simulink model "Full_Model_5"  (R2018b)
settings: Solver=VariableStepAuto  StartTime=0.0  StopTime=.5  RelTol=1e-3
InitFcn:
  | Robot_Body_Constants
values from neighbouring files (symbols this model uses):
  robot_radius = 0.0789    [Robot_Body_Constants.m]
  wheel_angles = [pi * 0.25 pi * 0.75 pi * 1.25 pi * 1.75]    [Robot_Body_Constants.m]
libraries: powerlib x56, peBldcCurrentController x4, simulink x1, dspinverses x1
(part 1 of 2)
settings Model: Creator=Zach  LastModifiedBy=Zach

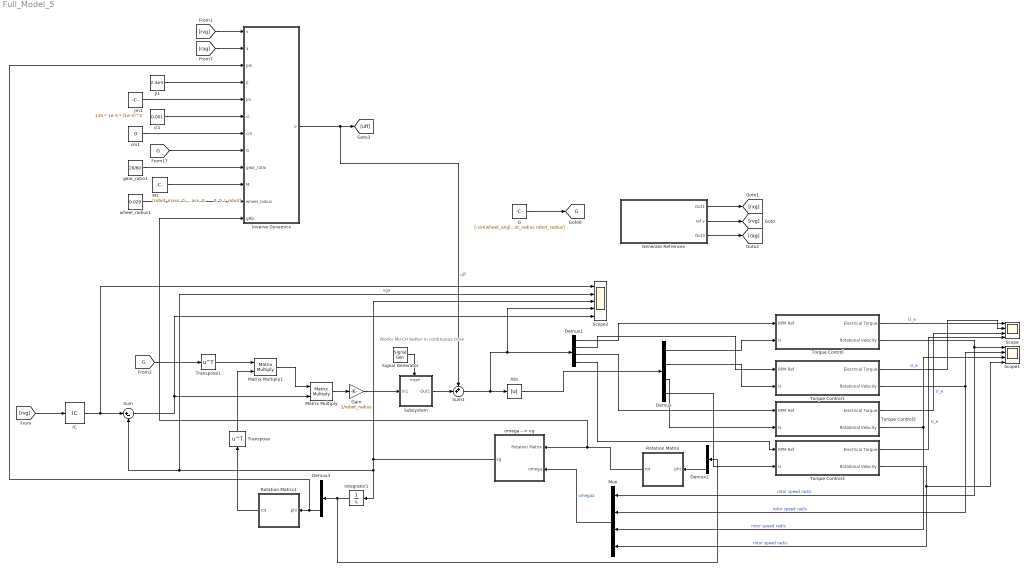
== system Full_Model_5 ==
  note: Works MUCH better in continuous time
  Abs : Abs
  Demux : Demux
  Demux1 : Demux
  Demux2 : Demux  Outputs=3
  Demux3 : Demux  Outputs=3
  G : Constant  Value=[-sin(wheel_angles(1)) -sin(wheel_angles(2)) -sin(wheel_angles(3)) -sin(wheel_angles(4)); cos(wheel_angles(1)) cos(wheel_angles(2)) cos(wheel_angles(3)) cos(wheel_angles(4)); robot_radius robot_radius robot_radius robot_radius]
  Gain : Gain  Gain=1/robot_radius
  Generate Refrences : Subsystem
  IC : InitialCondition  Value=[0;0;0]
  Integrator1 : Integrator
  Inverse Dynamics : MATLAB Function  TreatAsAtomicUnit=on
  Jl1 : Constant  Value=2.4e-5
  Jm1 : Constant  Value=135 * 1e-3 * (1e-2)^2
  M1 : Constant  Value=|
      | [robot_mass, 0, 0;
      |      0, robot_mass, 0;
      |      0, 0, I_robot]
  Matrix Multiply : Product  Multiplication=Matrix(*)
  Matrix Multiply1 : Product  Multiplication=Matrix(*)
  Mux : Mux
  Rotation Matrix : MATLAB Function  TreatAsAtomicUnit=on
  Rotation Matrix1 : MATLAB Function  TreatAsAtomicUnit=on
  Scope : Scope  NumInputPorts=4
  Scope1 : Scope  NumInputPorts=4
  Scope2 : Scope  NumInputPorts=5
  Signal Generator : SignalGenerator  Frequency=100000
  Subsystem : Subsystem
  Sum : Sum  Inputs=|+-
  Sum1 : Sum  Inputs=++|
  Torque Control : Subsystem
  Torque Control1 : Subsystem
  Torque Control2 : Subsystem
  Torque Control3 : Subsystem
  Transpose : Math  Operator=transpose  SaturateOnIntegerOverflow=on
  Transpose1 : Math  Operator=transpose  SaturateOnIntegerOverflow=on
  cl1 : Constant  Value=0.001
  cm1 : Constant  Value=0
  gear_ratio1 : Constant  Value=20/60
  omega --> vg : Subsystem
  wheel_radius1 : Constant  Value=0.029
  tag scope: G=global
  wires:
  Mux/1 -> omega --> vg/2(omega)  "omegaa"
  omega --> vg/1(vg) -> Scope2/3, Scope2/2, Sum/2, Integrator1/1  "vga"
  Generate Refrences/1(Out1) -> [rxg]
  Generate Refrences/2(ref v) -> [rvg]
  Generate Refrences/3(Out3) -> [rag]
  [rvg] -> IC/1
  Torque Control/2(Rotational Velocity) -> Mux/1, Scope1/1  "rotor speed rad/s"
  Torque Control/1(Electrical Torque) -> Scope/1  "U_e"
  Integrator1/1 -> Demux2/1, Demux3/1
  Demux2/3 -> Rotation Matrix/1(phi)
  G/1 -> [G]
  Rotation Matrix1/1(rot) -> Transpose/1
  [G] -> Transpose1/1
  Transpose/1 -> Matrix Multiply1/2
  IC/1 -> Scope2/1, Sum/1
  Sum/1 -> Scope2/5, Matrix Multiply/2
  Matrix Multiply1/1 -> Matrix Multiply/1
  Torque Control1/1(Electrical Torque) -> Scope/2  "U_e"
  Torque Control1/2(Rotational Velocity) -> Mux/2, Scope1/2  "rotor speed rad/s"
  Torque Control3/2(Rotational Velocity) -> Scope1/4, Mux/4  "rotor speed rad/s"
  Torque Control2/2(Rotational Velocity) -> Mux/3, Scope1/3  "rotor speed rad/s"
  Torque Control2/1(Electrical Torque) -> Scope/3  "U_e"
  Torque Control3/1(Electrical Torque) -> Scope/4  "U_e"
  Matrix Multiply/1 -> Gain/1
  Transpose1/1 -> Matrix Multiply1/1
  Abs/1 -> Demux/1
  Demux/4 -> Torque Control3/2(Is)
  Demux/1 -> Torque Control/2(Is)
  Demux/2 -> Torque Control1/2(Is)
  Demux/3 -> Torque Control2/2(Is)
  Demux1/1 -> Torque Control/1(RPM Ref)
  Demux1/2 -> Torque Control1/1(RPM Ref)
  Demux1/3 -> Torque Control2/1(RPM Ref)
  Demux1/4 -> Torque Control3/1(RPM Ref)
  gear_ratio1/1 -> Inverse Dynamics/9(gear_ratio)
  [G] -> Inverse Dynamics/8(G)
  Demux3/3 -> Inverse Dynamics/3(phi), Rotation Matrix1/1(phi)
  [rvg] -> Inverse Dynamics/1(v)
  cl1/1 -> Inverse Dynamics/6(cl)
  wheel_radius1/1 -> Inverse Dynamics/11(wheel_radius)
  cm1/1 -> Inverse Dynamics/7(cm)
  Inverse Dynamics/1(u) -> Sum1/1, [uff]  "uff"
  Jm1/1 -> Inverse Dynamics/5(Jm)
  [rag] -> Inverse Dynamics/2(a)
  Rotation Matrix/1(rot) -> Inverse Dynamics/12(gRb), omega --> vg/1(Rotation Matrix)
  Jl1/1 -> Inverse Dynamics/4(Jl)
  M1/1 -> Inverse Dynamics/10(M)
  Sum1/1 -> Scope2/4, Demux1/1, Abs/1
  Gain/1 -> Subsystem/1(In1)
  Subsystem/1(Out1) -> Sum1/2
  Signal Generator/1 -> Subsystem/Trigger

== system Full_Model_5/Generate Refrences ==
  Clock : Clock
  Constant : Constant  Value=3
  Gen Ref Values : MATLAB Function  TreatAsAtomicUnit=on
  Scope : Scope
  Out1 : Outport
  ref v : Outport  Port=2
  Out3 : Outport  Port=3
  wires:
  Clock/1 -> Scope/1, Gen Ref Values/2(t)
  Constant/1 -> Gen Ref Values/1(v)
  Gen Ref Values/1(rx) -> Out1/1
  Gen Ref Values/2(rv) -> ref v/1  "ref v"
  Gen Ref Values/3(ra) -> Out3/1

== system Full_Model_5/Subsystem ==
  In1 : Inport
  Trigger : TriggerPort  VariantControl=Variant  PortDimensions=1
  PID Controller : simulink/Continuous/PID Controller  Controller=PID  Form=Parallel  TimeDomain=Discrete-time  SampleTime=-1  IntegratorMethod=Forward Euler  FilterMethod=Forward Euler  ControllerParametersSource=internal  P=8  I=2  D=0  UseFilter=on  N=100  TunerSelectOption=Transfer Function Based (PID Tuner App)  InitialConditionSource=internal  InitialConditionForIntegrator=0  InitialConditionForFilter=0  DifferentiatorICPrevScaledInput=0  ExternalReset=none  TrackingMode=off  Kt=1  LimitOutput=on  UpperSaturationLimit=40  LowerSaturationLimit=-40  LinearizeAsGain=on  AntiWindupMode=none  Kb=1  POutMin=[]  POutMax=[]  IOutMin=[]  IOutMax=[]  DOutMin=[]  DOutMax=[]  NOutMin=[]  NOutMax=[]  SumOutMin=[]  SumOutMax=[]  SaturationOutMin=[]  SaturationOutMax=[]  PParamMin=[]  PParamMax=[]  IParamMin=[]  IParamMax=[]  DParamMin=[]  DParamMax=[]  NParamMin=[]  NParamMax=[]  KbParamMin=[]  KbParamMax=[]  KtParamMin=[]  KtParamMax=[]  KbOutMin=[]  KbOutMax=[]  KtOutMin=[]  KtOutMax=[]  IntegratorOutMin=[]  IntegratorOutMax=[]  FilterOutMin=[]  FilterOutMax=[]  SumI1OutMin=[]  SumI1OutMax=[]  SumI2OutMin=[]  SumI2OutMax=[]  SumI3OutMin=[]  SumI3OutMax=[]  SumI4OutMin=[]  SumI4OutMax=[]  SumDOutMin=[]  SumDOutMax=[]  DifferentiatorOutMin=[]  DifferentiatorOutMax=[]  FilterDiffOutCoefMin=[]  FilterDiffOutCoefMax=[]  ReciprocalOutMin=[]  ReciprocalOutMax=[]  SumDenOutMin=[]  SumDenOutMax=[]  SumNumOutMin=[]  SumNumOutMax=[]  DivideOutMin=[]  DivideOutMax=[]  IntegratorContinuousStateAttributes=''  IntegratorStateMustResolveToSignalObject=off  IntegratorRTWStateStorageClass=Auto  FilterContinuousStateAttributes=''  FilterStateMustResolveToSignalObject=off  FilterRTWStateStorageClass=Auto  ParallelPVariant=InternalParameters  IdealPVariant=Disabled  IVariant=InternalParameters  DVariant=InternalParameters  IntegratorVariant=Discrete  SatVariant=Enabled  AWVariant=Passthrough  PCopyVariant=Disabled  TRVariant=Disabled  FdbkBlocksVariant=Forward  IdealPFdbkVariant=Disabled  SatFdbkVariant=Disabled  DerivativeFilterVariant=ForwardEulerFilter  NVariant=InternalParameters  NCopyVariant=Disabled  FilterICVariant=InternalICsFilter  IntegratorICVariant=InternalICs  ExternalResetVariant=Disabled  TRSumVariant=Passthrough  SumFdbkVariant=Disabled  SumVariant=Sum_PID
  Out1 : Outport
  wires:
  In1/1 -> PID Controller/1
  PID Controller/1 -> Out1/1

== system Full_Model_5/Torque Control ==
  note: Needed for direction
  RPM Ref : Inport
  Is : Inport  Port=2
  Subsystem : Subsystem
  Subsystem1 : Subsystem
  Electrical Torque : Outport
  Rotational Velocity : Outport  Port=2
  wires:
  Subsystem/1(Gating Signals (PWM)) -> Subsystem1/1(Gating Signals)
  RPM Ref/1 -> Subsystem/1(rpm ref)
  Is/1 -> Subsystem/2(Is*)
  Subsystem1/2(Omega) -> Rotational Velocity/1
  Subsystem1/1(Te) -> Electrical Torque/1
  Subsystem1/3(Iabc) -> Subsystem/3(Iabc)
  Subsystem1/4(Out1) -> Subsystem/4(H1)
  Subsystem1/5(Out2) -> Subsystem/5(H2)
  Subsystem1/6(Out3) -> Subsystem/6(H3)

== system Full_Model_5/Torque Control1 ==
  note: Needed for direction
  RPM Ref : Inport
  Is : Inport  Port=2
  Subsystem : Subsystem
  Subsystem1 : Subsystem
  Electrical Torque : Outport
  Rotational Velocity : Outport  Port=2
  wires:
  Subsystem1/6(Out3) -> Subsystem/6(H3)
  Subsystem1/5(Out2) -> Subsystem/5(H2)
  Subsystem1/4(Out1) -> Subsystem/4(H1)
  Subsystem1/3(Iabc) -> Subsystem/3(Iabc)
  Subsystem1/1(Te) -> Electrical Torque/1
  Subsystem1/2(Omega) -> Rotational Velocity/1
  Is/1 -> Subsystem/2(Is*)
  RPM Ref/1 -> Subsystem/1(rpm ref)
  Subsystem/1(Gating Signals (PWM)) -> Subsystem1/1(Gating Signals)

== system Full_Model_5/Torque Control2 ==
  note: Needed for direction
  RPM Ref : Inport
  Is : Inport  Port=2
  Subsystem : Subsystem
  Subsystem1 : Subsystem
  Electrical Torque : Outport
  Rotational Velocity : Outport  Port=2
  wires:
  Subsystem/1(Gating Signals (PWM)) -> Subsystem1/1(Gating Signals)
  RPM Ref/1 -> Subsystem/1(rpm ref)
  Is/1 -> Subsystem/2(Is*)
  Subsystem1/2(Omega) -> Rotational Velocity/1
  Subsystem1/1(Te) -> Electrical Torque/1
  Subsystem1/3(Iabc) -> Subsystem/3(Iabc)
  Subsystem1/4(Out1) -> Subsystem/4(H1)
  Subsystem1/5(Out2) -> Subsystem/5(H2)
  Subsystem1/6(Out3) -> Subsystem/6(H3)

== system Full_Model_5/Torque Control3 ==
  note: Needed for direction
  RPM Ref : Inport
  Is : Inport  Port=2
  Subsystem : Subsystem
  Subsystem1 : Subsystem
  Electrical Torque : Outport
  Rotational Velocity : Outport  Port=2
  wires:
  Subsystem1/6(Out3) -> Subsystem/6(H3)
  Subsystem1/5(Out2) -> Subsystem/5(H2)
  Subsystem1/4(Out1) -> Subsystem/4(H1)
  Subsystem1/3(Iabc) -> Subsystem/3(Iabc)
  Subsystem1/1(Te) -> Electrical Torque/1
  Subsystem1/2(Omega) -> Rotational Velocity/1
  Is/1 -> Subsystem/2(Is*)
  RPM Ref/1 -> Subsystem/1(rpm ref)
  Subsystem/1(Gating Signals (PWM)) -> Subsystem1/1(Gating Signals)

== system Full_Model_5/omega --> vg ==
  Rotation Matrix : Inport
  omega : Inport  Port=2
  Gain : Gain  Gain=robot_radius
  Matrix Multiply : Product  Inputs=3  Multiplication=Matrix(*)
  Pseudoinverse : dspinverses/Pseudoinverse  wanterr=off  SimulateUsing=Interpreted execution
      settings: SourceProductName=DSP System Toolbox  SourceProductBaseCode=DS
  Transpose : Math  Operator=transpose  SaturateOnIntegerOverflow=on
  vg : Outport
  wires:
  [G] -> Transpose/1
  Transpose/1 -> Pseudoinverse/1
  omega/1 -> Matrix Multiply/3
  Matrix Multiply/1 -> Gain/1
  Gain/1 -> vg/1
  Pseudoinverse/1 -> Matrix Multiply/2
  Rotation Matrix/1 -> Matrix Multiply/1

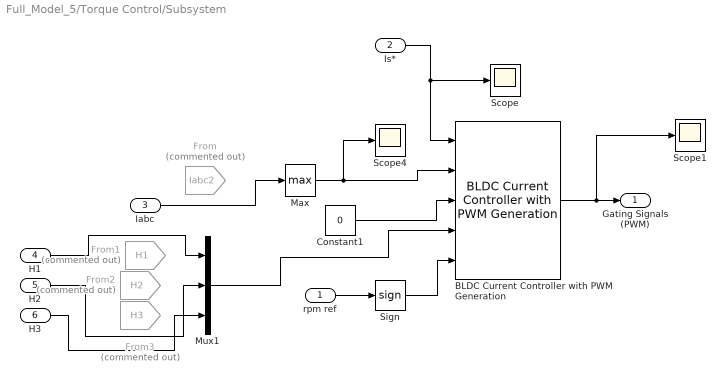
== system Full_Model_5/Torque Control/Subsystem ==
  rpm ref : Inport
  Is* : Inport  Port=2
  Iabc : Inport  Port=3
  H1 : Inport  Port=4
  H2 : Inport  Port=5
  H3 : Inport  Port=6
  BLDC Current Controller with PWM Generation : peBldcCurrentController/BLDC Current Controller with PWM Generation  Kp=40  Ki=10  Kaw=100  Ts=-1  Tsd=0.001  ActZC=off  CarrCount=Up  Tper=.0001  Tfundamental=.00001
  Constant1 : Constant  Value=0
  From : From  Commented=on  GotoTag=Iabc2  TagVisibility=global
  From1 : From  Commented=on  GotoTag=H1  TagVisibility=global
  From2 : From  Commented=on  GotoTag=H2  TagVisibility=global
  From3 : From  Commented=on  GotoTag=H3  TagVisibility=global
  Max : MinMax  Function=max
  Mux1 : Mux  Inputs=3
  Scope : Scope
  Scope1 : Scope
  Scope4 : Scope
  Sign : Signum
  Gating Signals (PWM) : Outport
  wires:
  rpm ref/1 -> Sign/1
  Mux1/1 -> BLDC Current Controller with PWM Generation/4
  Sign/1 -> BLDC Current Controller with PWM Generation/5
  Constant1/1 -> BLDC Current Controller with PWM Generation/3
  Max/1 -> BLDC Current Controller with PWM Generation/2, Scope4/1
  BLDC Current Controller with PWM Generation/1 -> Scope1/1, Gating Signals (PWM)/1
  Is*/1 -> Scope/1, BLDC Current Controller with PWM Generation/1
  Iabc/1 -> Max/1
  H1/1 -> Mux1/1
  H2/1 -> Mux1/2
  H3/1 -> Mux1/3

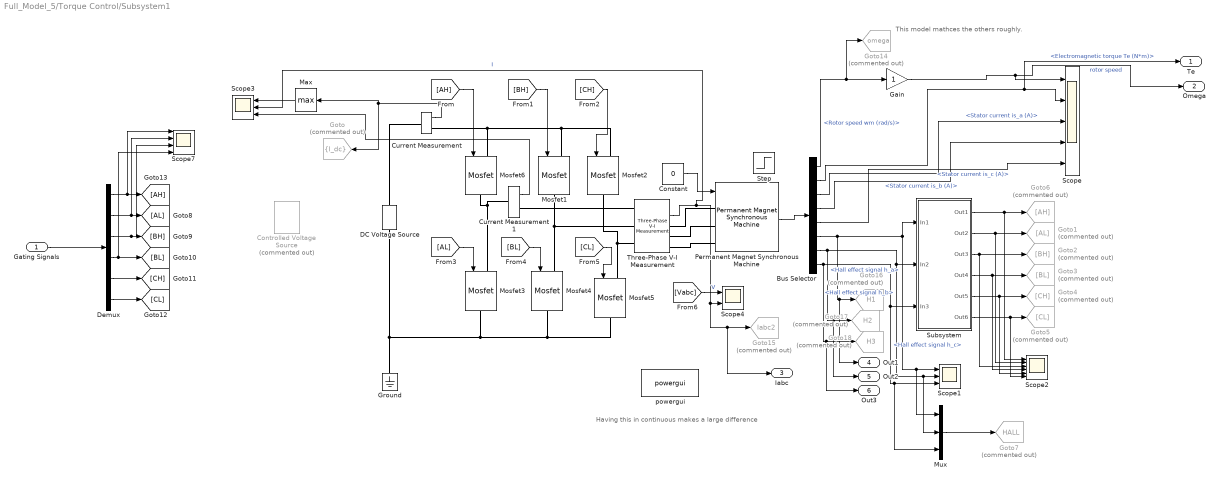
== system Full_Model_5/Torque Control/Subsystem1 ==
  note: This model mathces the others roughly.
  note: Having this in continuous makes a large difference
  Gating Signals : Inport
  Bus Selector : BusSelector  OutputSignals=Rotor speed wm (rad/s),Electromagnetic torque Te (N*m),Stator current is_a (A),Stator current is_b (A),Stator current is_c (A),Hall effect signal h_a,Hall effect signal h_b,Hall effect signal h_c
  Constant : Constant  Value=0
  Controlled Voltage Source : powerlib/Electrical Sources/Controlled Voltage Source  Commented=on  Initialize=off  Source_Type=DC  Amplitude=24  Phase=0  Frequency=0  Measurements=Voltage
  Current Measurement : powerlib/Measurements/Current Measurement  PhasorSimulation=off  OutputType=Magnitude  PSBequivalent=0
  Current Measurement1 : powerlib/Measurements/Current Measurement  PhasorSimulation=off  OutputType=Complex  PSBequivalent=0
  DC Voltage Source : powerlib/Electrical Sources/DC Voltage Source  Amplitude=24  Measurements=None
  Demux : Demux  Outputs=6
  Gain : Gain
  Goto : Goto  Commented=on  GotoTag=I_dc  TagVisibility=scoped
  Goto1 : Goto  Commented=on  GotoTag=AL
  Goto14 : Goto  Commented=on  GotoTag=omega  TagVisibility=global
  Goto15 : Goto  Commented=on  GotoTag=Iabc2  TagVisibility=global
  Goto16 : Goto  Commented=on  GotoTag=H1  TagVisibility=global
  Goto17 : Goto  Commented=on  GotoTag=H2  TagVisibility=global
  Goto18 : Goto  Commented=on  GotoTag=H3  TagVisibility=global
  Goto2 : Goto  Commented=on  GotoTag=BH
  Goto3 : Goto  Commented=on  GotoTag=BL
  Goto4 : Goto  Commented=on  GotoTag=CH
  Goto5 : Goto  Commented=on  GotoTag=CL
  Goto6 : Goto  Commented=on  GotoTag=AH
  Goto7 : Goto  Commented=on  GotoTag=HALL  TagVisibility=global
  Ground : powerlib/Elements/Ground  LConnTagsString=a
  Max : MinMax  Function=max
  Mosfet{1..6} (6 alike) : powerlib/Power Electronics/Mosfet  Ron=0.1  Lon=0  Rd=0.01  Vfd=0  IC=0  Rs=1e5  Cs=inf  Measurements=off
  Mux : Mux  Inputs=3
  Permanent Magnet Synchronous Machine : powerlib/Machines/Permanent Magnet Synchronous Machine  NbPhases=3  FluxDistribution=Trapezoidal  RotorType=Round  MechanicalLoad=Torque Tm  PresetModel=No  ShowDetailedParameters=on  MeasurementBus=off  Resistance=0.304  Inductance=0.0002315  dqInductances=[8.5e-3,8.5e-3]  La=0.0002315  MachineConstant=Torque Constant (N.m / A_peak)  Flux=0.003258  VoltageCst=5.4588  TorqueCst=0.052128  Flat=120  Mechanical=[1.81e-05 1e-07 8]  PolePairs=4  InitialConditions=[0,0, 0,0]  InitialConditions5ph=[0 0 0 0 0 0]  TsPowergui=0  TsBlock=-1  RefAngle=Aligned with phase A axis (original Park)
      settings: SourceProductName=Simscape Power Systems
  Scope : Scope  NumInputPorts=5
  Scope1 : Scope  NumInputPorts=3
  Scope2 : Scope  NumInputPorts=6
  Scope3 : Scope  NumInputPorts=3
  Scope4 : Scope  NumInputPorts=2
  Scope7 : Scope  NumInputPorts=4
  Step : Step  Time=.1  After=.125  SampleTime=0
  Subsystem : Subsystem
  Three-Phase V-I Measurement : powerlib/Measurements/Three-Phase V-I Measurement  VoltageMeasurement=phase-to-ground  SetLabelV=off  LabelV=Vabc  Vpu=off  VpuLL=off  CurrentMeasurement=yes  SetLabelI=off  LabelI=Iabc  Ipu=off  Pbase=100e6  Vbase=500e3  OutputType=Complex  PhasorSimulation=off  PSBequivalent=0
  powergui : powerlib/powergui  Priority=1  SimulationMode=Continuous  SampleTime=50e-6  frequency=60  Iterations=50  frequencyindice=0  Pbase=100e6  ErrMax=1e-4  UnitsV=kV  UnitsW=MW  buscounter=0  FunctionMessages=off  echomessages=off  EnableUseOfTLC=off  CurrentSourceSwitches=off  DisableSnubberDevices=off  DisableRonSwitches=off  DisableVfSwitches=off  DisplayEquations=off  SolverType=Tustin/Backward Euler (TBE)  Interpol=off  ExternalGateDelay=off  methode=off  Ts=100  x0status=blocks  SPID=on  SwTol=0  HookPort=off  RestoreLinks=warning  ResistiveCurrentMeasurement=off  Frange=[0:2:500]  Ylog=off  Xlog=on  ShowGrid=off  save=off  variable=ZData  structure=0  ZoomFFT=off  StartTime=0.0  cycles=1  DisplayStyle=1  fundamental=60  FreqAxis=off  MaxFrequency=1000  frequencyindicesteady=1  RmsSteady=1  display=off
  Te : Outport
  Omega : Outport  Port=2
  Iabc : Outport  Port=3
  Out1 : Outport  Port=4
  Out2 : Outport  Port=5
  Out3 : Outport  Port=6
  wires:
  [CH] -> Mosfet2/1
  Subsystem/6(Out6) -> Scope2/6, Goto5/1
  Subsystem/2(Out2) -> Scope2/2, Goto1/1
  Bus Selector/8 -> Out3/1, Goto18/1, Mux/3, Scope1/3, Subsystem/3(In3)  "<Hall effect signal h_c>"
  Subsystem/1(Out1) -> Scope2/1, Goto6/1
  Subsystem/3(Out3) -> Scope2/3, Goto2/1
  Bus Selector/2 -> Te/1, Scope/2  "<Electromagnetic torque Te (N*m)>"
  Subsystem/4(Out4) -> Scope2/4, Goto3/1
  Bus Selector/1 -> Goto14/1, Gain/1  "<Rotor speed wm (rad/s)>"
  Bus Selector/7 -> Out2/1, Goto17/1, Mux/2, Scope1/2, Subsystem/2(In2)  "<Hall effect signal h_b>"
  Mux/1 -> Goto7/1
  [AL] -> Mosfet3/1
  [BL] -> Mosfet4/1
  Bus Selector/6 -> Out1/1, Goto16/1, Subsystem/1(In1), Mux/1, Scope1/1  "<Hall effect signal h_a>"
  Subsystem/5(Out5) -> Scope2/5, Goto4/1
  [CL] -> Mosfet5/1
  Current Measurement/1 -> Max/1, Goto/1
  Bus Selector/3 -> Scope/3  "<Stator current is_a (A)>"
  Permanent Magnet Synchronous Machine/1 -> Bus Selector/1
  [BH] -> Mosfet1/1
  [AH] -> Mosfet6/1
  Bus Selector/4 -> Scope/4  "<Stator current is_b (A)>"
  Gain/1 -> Omega/1, Scope/1  "rotor speed"
  Bus Selector/5 -> Scope/5  "<Stator current is_c (A)>"
  Demux/6 -> [CL]
  Demux/5 -> [CH]
  Demux/4 -> [BL], Scope7/4
  Demux/3 -> Scope7/3, [BH]
  Demux/2 -> Scope7/2, [AL]
  Demux/1 -> Scope7/1, [AH]
  [Vabc] -> Scope4/1  "V"
  Three-Phase V-I Measurement/2 -> Iabc/1, Goto15/1, Scope4/2, Scope3/2  "I"
  Gating Signals/1 -> Demux/1
  Max/1 -> Scope3/1
  Current Measurement1/1 -> Scope3/3
  Constant/1 -> Permanent Magnet Synchronous Machine/1
  connections:
  Mosfet1/RConn1 -- Three-Phase V-I Measurement/LConn2 -- Mosfet4/LConn1
  Mosfet2/RConn1 -- Three-Phase V-I Measurement/LConn3 -- Mosfet5/LConn1
  Mosfet6/RConn1 -- Current Measurement1/LConn1 -- Mosfet3/LConn1
  Mosfet6/LConn1 -- Current Measurement/RConn1 -- Mosfet2/LConn1 -- Mosfet1/LConn1
  Ground/LConn1 -- DC Voltage Source/LConn1 -- Mosfet5/RConn1 -- Mosfet4/RConn1 -- Mosfet3/RConn1
  Three-Phase V-I Measurement/RConn1 -- Permanent Magnet Synchronous Machine/LConn1
  Three-Phase V-I Measurement/RConn2 -- Permanent Magnet Synchronous Machine/LConn2
  Permanent Magnet Synchronous Machine/LConn3 -- Three-Phase V-I Measurement/RConn3
  DC Voltage Source/RConn1 -- Current Measurement/LConn1
  Current Measurement1/RConn1 -- Three-Phase V-I Measurement/LConn1

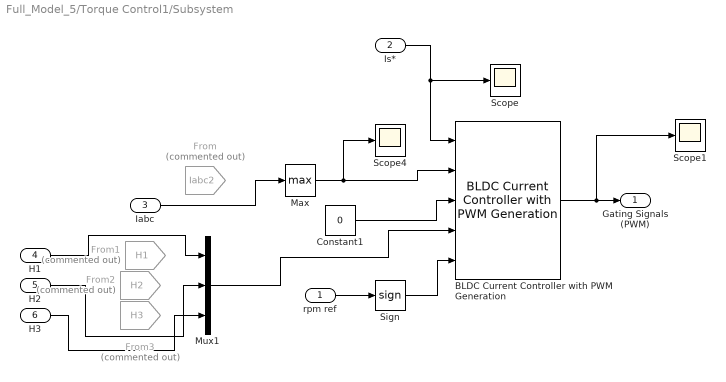
== system Full_Model_5/Torque Control1/Subsystem ==
  rpm ref : Inport
  Is* : Inport  Port=2
  Iabc : Inport  Port=3
  H1 : Inport  Port=4
  H2 : Inport  Port=5
  H3 : Inport  Port=6
  BLDC Current Controller with PWM Generation : peBldcCurrentController/BLDC Current Controller with PWM Generation  Kp=40  Ki=10  Kaw=100  Ts=-1  Tsd=0.001  ActZC=off  CarrCount=Up  Tper=.0001  Tfundamental=.00001
  Constant1 : Constant  Value=0
  From : From  Commented=on  GotoTag=Iabc2  TagVisibility=global
  From1 : From  Commented=on  GotoTag=H1  TagVisibility=global
  From2 : From  Commented=on  GotoTag=H2  TagVisibility=global
  From3 : From  Commented=on  GotoTag=H3  TagVisibility=global
  Max : MinMax  Function=max
  Mux1 : Mux  Inputs=3
  Scope : Scope
  Scope1 : Scope
  Scope4 : Scope
  Sign : Signum
  Gating Signals (PWM) : Outport
  wires:
  H3/1 -> Mux1/3
  H2/1 -> Mux1/2
  H1/1 -> Mux1/1
  Iabc/1 -> Max/1
  Is*/1 -> BLDC Current Controller with PWM Generation/1, Scope/1
  BLDC Current Controller with PWM Generation/1 -> Gating Signals (PWM)/1, Scope1/1
  Max/1 -> Scope4/1, BLDC Current Controller with PWM Generation/2
  Constant1/1 -> BLDC Current Controller with PWM Generation/3
  Sign/1 -> BLDC Current Controller with PWM Generation/5
  Mux1/1 -> BLDC Current Controller with PWM Generation/4
  rpm ref/1 -> Sign/1

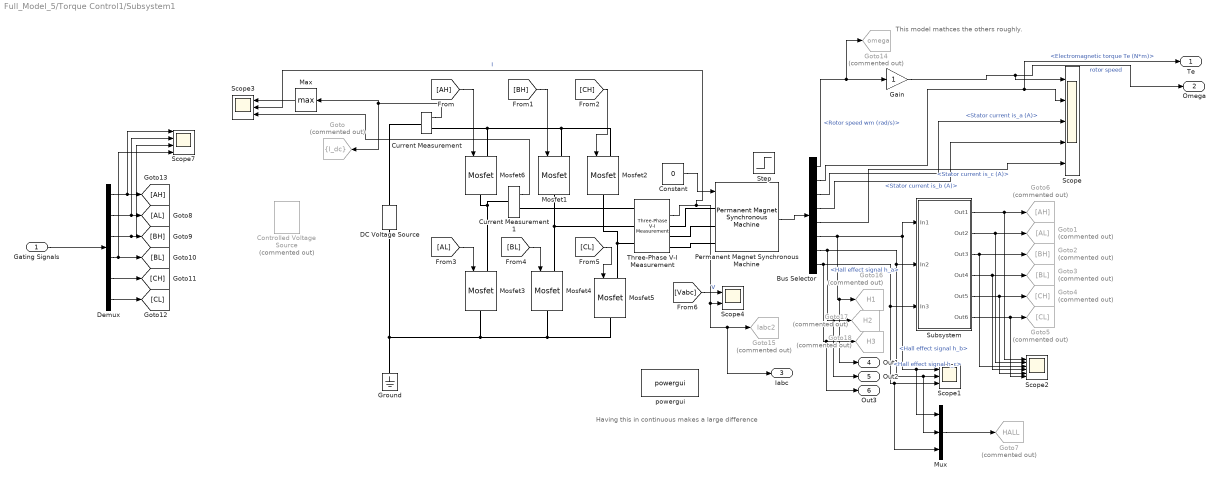
== system Full_Model_5/Torque Control1/Subsystem1 ==
  note: Having this in continuous makes a large difference
  note: This model mathces the others roughly.
  Gating Signals : Inport
  Bus Selector : BusSelector  OutputSignals=Rotor speed wm (rad/s),Electromagnetic torque Te (N*m),Stator current is_a (A),Stator current is_b (A),Stator current is_c (A),Hall effect signal h_a,Hall effect signal h_b,Hall effect signal h_c
  Constant : Constant  Value=0
  Controlled Voltage Source : powerlib/Electrical Sources/Controlled Voltage Source  Commented=on  Initialize=off  Source_Type=DC  Amplitude=24  Phase=0  Frequency=0  Measurements=Voltage
  Current Measurement : powerlib/Measurements/Current Measurement  PhasorSimulation=off  OutputType=Magnitude  PSBequivalent=0
  Current Measurement1 : powerlib/Measurements/Current Measurement  PhasorSimulation=off  OutputType=Complex  PSBequivalent=0
  DC Voltage Source : powerlib/Electrical Sources/DC Voltage Source  Amplitude=24  Measurements=None
  Demux : Demux  Outputs=6
  Gain : Gain
  Goto : Goto  Commented=on  GotoTag=I_dc  TagVisibility=scoped
  Goto1 : Goto  Commented=on  GotoTag=AL
  Goto14 : Goto  Commented=on  GotoTag=omega  TagVisibility=global
  Goto15 : Goto  Commented=on  GotoTag=Iabc2  TagVisibility=global
  Goto16 : Goto  Commented=on  GotoTag=H1  TagVisibility=global
  Goto17 : Goto  Commented=on  GotoTag=H2  TagVisibility=global
  Goto18 : Goto  Commented=on  GotoTag=H3  TagVisibility=global
  Goto2 : Goto  Commented=on  GotoTag=BH
  Goto3 : Goto  Commented=on  GotoTag=BL
  Goto4 : Goto  Commented=on  GotoTag=CH
  Goto5 : Goto  Commented=on  GotoTag=CL
  Goto6 : Goto  Commented=on  GotoTag=AH
  Goto7 : Goto  Commented=on  GotoTag=HALL  TagVisibility=global
  Ground : powerlib/Elements/Ground  LConnTagsString=a
  Max : MinMax  Function=max
  Mosfet{1..6} (6 alike) : powerlib/Power Electronics/Mosfet  Ron=0.1  Lon=0  Rd=0.01  Vfd=0  IC=0  Rs=1e5  Cs=inf  Measurements=off
  Mux : Mux  Inputs=3
  Permanent Magnet Synchronous Machine : powerlib/Machines/Permanent Magnet Synchronous Machine  NbPhases=3  FluxDistribution=Trapezoidal  RotorType=Round  MechanicalLoad=Torque Tm  PresetModel=No  ShowDetailedParameters=on  MeasurementBus=off  Resistance=0.304  Inductance=0.0002315  dqInductances=[8.5e-3,8.5e-3]  La=0.0002315  MachineConstant=Torque Constant (N.m / A_peak)  Flux=0.003258  VoltageCst=5.4588  TorqueCst=0.052128  Flat=120  Mechanical=[1.81e-05 1e-07 8]  PolePairs=4  InitialConditions=[0,0, 0,0]  InitialConditions5ph=[0 0 0 0 0 0]  TsPowergui=0  TsBlock=-1  RefAngle=Aligned with phase A axis (original Park)
      settings: SourceProductName=Simscape Power Systems
  Scope : Scope  NumInputPorts=5
  Scope1 : Scope  NumInputPorts=3
  Scope2 : Scope  NumInputPorts=6
  Scope3 : Scope  NumInputPorts=3
  Scope4 : Scope  NumInputPorts=2
  Scope7 : Scope  NumInputPorts=4
  Step : Step  Time=.1  After=.125  SampleTime=0
  Subsystem : Subsystem
  Three-Phase V-I Measurement : powerlib/Measurements/Three-Phase V-I Measurement  VoltageMeasurement=phase-to-ground  SetLabelV=off  LabelV=Vabc  Vpu=off  VpuLL=off  CurrentMeasurement=yes  SetLabelI=off  LabelI=Iabc  Ipu=off  Pbase=100e6  Vbase=500e3  OutputType=Complex  PhasorSimulation=off  PSBequivalent=0
  powergui : powerlib/powergui  Priority=1  SimulationMode=Continuous  SampleTime=50e-6  frequency=60  Iterations=50  frequencyindice=0  Pbase=100e6  ErrMax=1e-4  UnitsV=kV  UnitsW=MW  buscounter=0  FunctionMessages=off  echomessages=off  EnableUseOfTLC=off  CurrentSourceSwitches=off  DisableSnubberDevices=off  DisableRonSwitches=off  DisableVfSwitches=off  DisplayEquations=off  SolverType=Tustin/Backward Euler (TBE)  Interpol=off  ExternalGateDelay=off  methode=off  Ts=100  x0status=blocks  SPID=on  SwTol=0  HookPort=off  RestoreLinks=warning  ResistiveCurrentMeasurement=off  Frange=[0:2:500]  Ylog=off  Xlog=on  ShowGrid=off  save=off  variable=ZData  structure=0  ZoomFFT=off  StartTime=0.0  cycles=1  DisplayStyle=1  fundamental=60  FreqAxis=off  MaxFrequency=1000  frequencyindicesteady=1  RmsSteady=1  display=off
  Te : Outport
  Omega : Outport  Port=2
  Iabc : Outport  Port=3
  Out1 : Outport  Port=4
  Out2 : Outport  Port=5
  Out3 : Outport  Port=6
  wires:
  Constant/1 -> Permanent Magnet Synchronous Machine/1
  Current Measurement1/1 -> Scope3/3
  Max/1 -> Scope3/1
  Gating Signals/1 -> Demux/1
  Three-Phase V-I Measurement/2 -> Scope3/2, Scope4/2, Goto15/1, Iabc/1  "I"
  [Vabc] -> Scope4/1  "V"
  Demux/1 -> [AH], Scope7/1
  Demux/2 -> [AL], Scope7/2
  Demux/3 -> [BH], Scope7/3
  Demux/4 -> Scope7/4, [BL]
  Demux/5 -> [CH]
  Demux/6 -> [CL]
  Bus Selector/5 -> Scope/5  "<Stator current is_c (A)>"
  Gain/1 -> Scope/1, Omega/1  "rotor speed"
  Bus Selector/4 -> Scope/4  "<Stator current is_b (A)>"
  [AH] -> Mosfet6/1
  [BH] -> Mosfet1/1
  Permanent Magnet Synchronous Machine/1 -> Bus Selector/1
  Bus Selector/3 -> Scope/3  "<Stator current is_a (A)>"
  Current Measurement/1 -> Goto/1, Max/1
  [CL] -> Mosfet5/1
  Subsystem/5(Out5) -> Goto4/1, Scope2/5
  Bus Selector/6 -> Scope1/1, Mux/1, Subsystem/1(In1), Goto16/1, Out1/1  "<Hall effect signal h_a>"
  [BL] -> Mosfet4/1
  [AL] -> Mosfet3/1
  Mux/1 -> Goto7/1
  Bus Selector/7 -> Subsystem/2(In2), Scope1/2, Mux/2, Goto17/1, Out2/1  "<Hall effect signal h_b>"
  Bus Selector/1 -> Gain/1, Goto14/1  "<Rotor speed wm (rad/s)>"
  Subsystem/4(Out4) -> Goto3/1, Scope2/4
  Bus Selector/2 -> Scope/2, Te/1  "<Electromagnetic torque Te (N*m)>"
  Subsystem/3(Out3) -> Goto2/1, Scope2/3
  Subsystem/1(Out1) -> Goto6/1, Scope2/1
  Bus Selector/8 -> Subsystem/3(In3), Scope1/3, Mux/3, Goto18/1, Out3/1  "<Hall effect signal h_c>"
  Subsystem/2(Out2) -> Goto1/1, Scope2/2
  Subsystem/6(Out6) -> Goto5/1, Scope2/6
  [CH] -> Mosfet2/1
  connections:
  Current Measurement1/RConn1 -- Three-Phase V-I Measurement/LConn1
  DC Voltage Source/RConn1 -- Current Measurement/LConn1
  Permanent Magnet Synchronous Machine/LConn3 -- Three-Phase V-I Measurement/RConn3
  Three-Phase V-I Measurement/RConn2 -- Permanent Magnet Synchronous Machine/LConn2
  Three-Phase V-I Measurement/RConn1 -- Permanent Magnet Synchronous Machine/LConn1
  Mosfet3/RConn1 -- Mosfet4/RConn1 -- Mosfet5/RConn1 -- DC Voltage Source/LConn1 -- Ground/LConn1
  Mosfet1/LConn1 -- Mosfet2/LConn1 -- Current Measurement/RConn1 -- Mosfet6/LConn1
  Mosfet3/LConn1 -- Current Measurement1/LConn1 -- Mosfet6/RConn1
  Mosfet5/LConn1 -- Three-Phase V-I Measurement/LConn3 -- Mosfet2/RConn1
  Mosfet4/LConn1 -- Three-Phase V-I Measurement/LConn2 -- Mosfet1/RConn1

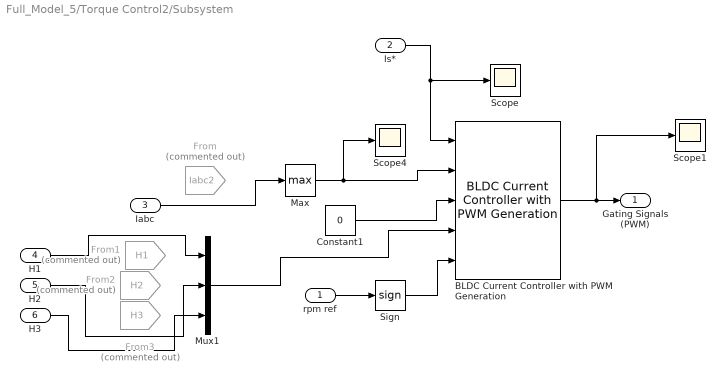
== system Full_Model_5/Torque Control2/Subsystem ==
  rpm ref : Inport
  Is* : Inport  Port=2
  Iabc : Inport  Port=3
  H1 : Inport  Port=4
  H2 : Inport  Port=5
  H3 : Inport  Port=6
  BLDC Current Controller with PWM Generation : peBldcCurrentController/BLDC Current Controller with PWM Generation  Kp=40  Ki=10  Kaw=100  Ts=-1  Tsd=0.001  ActZC=off  CarrCount=Up  Tper=.0001  Tfundamental=.00001
  Constant1 : Constant  Value=0
  From : From  Commented=on  GotoTag=Iabc2  TagVisibility=global
  From1 : From  Commented=on  GotoTag=H1  TagVisibility=global
  From2 : From  Commented=on  GotoTag=H2  TagVisibility=global
  From3 : From  Commented=on  GotoTag=H3  TagVisibility=global
  Max : MinMax  Function=max
  Mux1 : Mux  Inputs=3
  Scope : Scope
  Scope1 : Scope
  Scope4 : Scope
  Sign : Signum
  Gating Signals (PWM) : Outport
  wires:
  rpm ref/1 -> Sign/1
  Mux1/1 -> BLDC Current Controller with PWM Generation/4
  Sign/1 -> BLDC Current Controller with PWM Generation/5
  Constant1/1 -> BLDC Current Controller with PWM Generation/3
  Max/1 -> BLDC Current Controller with PWM Generation/2, Scope4/1
  BLDC Current Controller with PWM Generation/1 -> Scope1/1, Gating Signals (PWM)/1
  Is*/1 -> Scope/1, BLDC Current Controller with PWM Generation/1
  Iabc/1 -> Max/1
  H1/1 -> Mux1/1
  H2/1 -> Mux1/2
  H3/1 -> Mux1/3

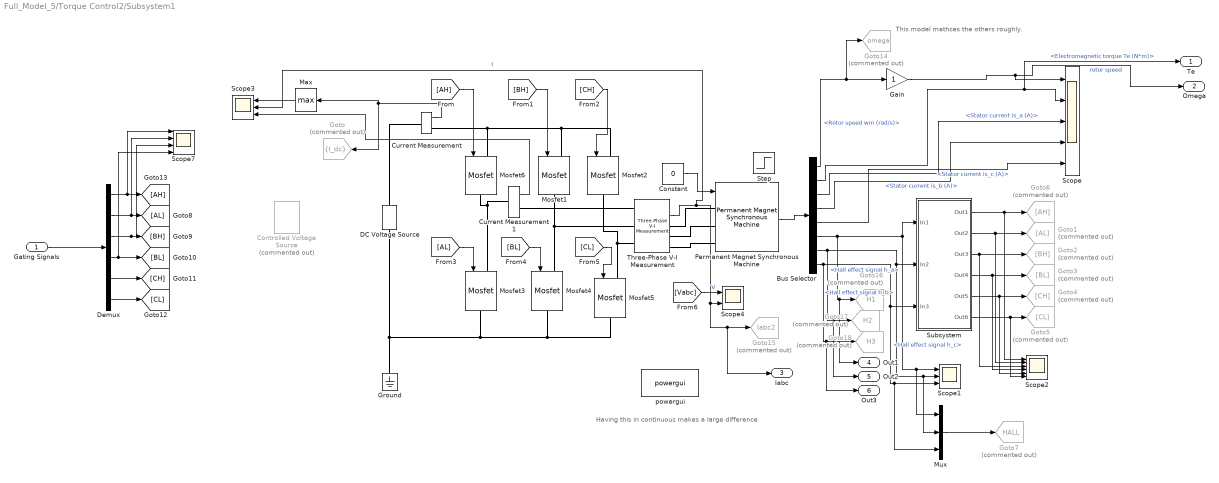
== system Full_Model_5/Torque Control2/Subsystem1 ==
  note: This model mathces the others roughly.
  note: Having this in continuous makes a large difference
  Gating Signals : Inport
  Bus Selector : BusSelector  OutputSignals=Rotor speed wm (rad/s),Electromagnetic torque Te (N*m),Stator current is_a (A),Stator current is_b (A),Stator current is_c (A),Hall effect signal h_a,Hall effect signal h_b,Hall effect signal h_c
  Constant : Constant  Value=0
  Controlled Voltage Source : powerlib/Electrical Sources/Controlled Voltage Source  Commented=on  Initialize=off  Source_Type=DC  Amplitude=24  Phase=0  Frequency=0  Measurements=Voltage
  Current Measurement : powerlib/Measurements/Current Measurement  PhasorSimulation=off  OutputType=Magnitude  PSBequivalent=0
  Current Measurement1 : powerlib/Measurements/Current Measurement  PhasorSimulation=off  OutputType=Complex  PSBequivalent=0
  DC Voltage Source : powerlib/Electrical Sources/DC Voltage Source  Amplitude=24  Measurements=None
  Demux : Demux  Outputs=6
  Gain : Gain
  Goto : Goto  Commented=on  GotoTag=I_dc  TagVisibility=scoped
  Goto1 : Goto  Commented=on  GotoTag=AL
  Goto14 : Goto  Commented=on  GotoTag=omega  TagVisibility=global
  Goto15 : Goto  Commented=on  GotoTag=Iabc2  TagVisibility=global
  Goto16 : Goto  Commented=on  GotoTag=H1  TagVisibility=global
  Goto17 : Goto  Commented=on  GotoTag=H2  TagVisibility=global
  Goto18 : Goto  Commented=on  GotoTag=H3  TagVisibility=global
  Goto2 : Goto  Commented=on  GotoTag=BH
  Goto3 : Goto  Commented=on  GotoTag=BL
  Goto4 : Goto  Commented=on  GotoTag=CH
  Goto5 : Goto  Commented=on  GotoTag=CL
  Goto6 : Goto  Commented=on  GotoTag=AH
  Goto7 : Goto  Commented=on  GotoTag=HALL  TagVisibility=global
  Ground : powerlib/Elements/Ground  LConnTagsString=a
  Max : MinMax  Function=max
  Mosfet{1..6} (6 alike) : powerlib/Power Electronics/Mosfet  Ron=0.1  Lon=0  Rd=0.01  Vfd=0  IC=0  Rs=1e5  Cs=inf  Measurements=off
  Mux : Mux  Inputs=3
  Permanent Magnet Synchronous Machine : powerlib/Machines/Permanent Magnet Synchronous Machine  NbPhases=3  FluxDistribution=Trapezoidal  RotorType=Round  MechanicalLoad=Torque Tm  PresetModel=No  ShowDetailedParameters=on  MeasurementBus=off  Resistance=0.304  Inductance=0.0002315  dqInductances=[8.5e-3,8.5e-3]  La=0.0002315  MachineConstant=Torque Constant (N.m / A_peak)  Flux=0.003258  VoltageCst=5.4588  TorqueCst=0.052128  Flat=120  Mechanical=[1.81e-05 1e-07 8]  PolePairs=4  InitialConditions=[0,0, 0,0]  InitialConditions5ph=[0 0 0 0 0 0]  TsPowergui=0  TsBlock=-1  RefAngle=Aligned with phase A axis (original Park)
      settings: SourceProductName=Simscape Power Systems
  Scope : Scope  NumInputPorts=5
  Scope1 : Scope  NumInputPorts=3
  Scope2 : Scope  NumInputPorts=6
  Scope3 : Scope  NumInputPorts=3
  Scope4 : Scope  NumInputPorts=2
  Scope7 : Scope  NumInputPorts=4
  Step : Step  Time=.1  After=.125  SampleTime=0
  Subsystem : Subsystem
  Three-Phase V-I Measurement : powerlib/Measurements/Three-Phase V-I Measurement  VoltageMeasurement=phase-to-ground  SetLabelV=off  LabelV=Vabc  Vpu=off  VpuLL=off  CurrentMeasurement=yes  SetLabelI=off  LabelI=Iabc  Ipu=off  Pbase=100e6  Vbase=500e3  OutputType=Complex  PhasorSimulation=off  PSBequivalent=0
  powergui : powerlib/powergui  Priority=1  SimulationMode=Continuous  SampleTime=50e-6  frequency=60  Iterations=50  frequencyindice=0  Pbase=100e6  ErrMax=1e-4  UnitsV=kV  UnitsW=MW  buscounter=0  FunctionMessages=off  echomessages=off  EnableUseOfTLC=off  CurrentSourceSwitches=off  DisableSnubberDevices=off  DisableRonSwitches=off  DisableVfSwitches=off  DisplayEquations=off  SolverType=Tustin/Backward Euler (TBE)  Interpol=off  ExternalGateDelay=off  methode=off  Ts=100  x0status=blocks  SPID=on  SwTol=0  HookPort=off  RestoreLinks=warning  ResistiveCurrentMeasurement=off  Frange=[0:2:500]  Ylog=off  Xlog=on  ShowGrid=off  save=off  variable=ZData  structure=0  ZoomFFT=off  StartTime=0.0  cycles=1  DisplayStyle=1  fundamental=60  FreqAxis=off  MaxFrequency=1000  frequencyindicesteady=1  RmsSteady=1  display=off
  Te : Outport
  Omega : Outport  Port=2
  Iabc : Outport  Port=3
  Out1 : Outport  Port=4
  Out2 : Outport  Port=5
  Out3 : Outport  Port=6
  wires:
  [CH] -> Mosfet2/1
  Subsystem/6(Out6) -> Scope2/6, Goto5/1
  Subsystem/2(Out2) -> Scope2/2, Goto1/1
  Bus Selector/8 -> Out3/1, Goto18/1, Mux/3, Scope1/3, Subsystem/3(In3)  "<Hall effect signal h_c>"
  Subsystem/1(Out1) -> Scope2/1, Goto6/1
  Subsystem/3(Out3) -> Scope2/3, Goto2/1
  Bus Selector/2 -> Te/1, Scope/2  "<Electromagnetic torque Te (N*m)>"
  Subsystem/4(Out4) -> Scope2/4, Goto3/1
  Bus Selector/1 -> Goto14/1, Gain/1  "<Rotor speed wm (rad/s)>"
  Bus Selector/7 -> Out2/1, Goto17/1, Mux/2, Scope1/2, Subsystem/2(In2)  "<Hall effect signal h_b>"
  Mux/1 -> Goto7/1
  [AL] -> Mosfet3/1
  [BL] -> Mosfet4/1
  Bus Selector/6 -> Out1/1, Goto16/1, Subsystem/1(In1), Mux/1, Scope1/1  "<Hall effect signal h_a>"
  Subsystem/5(Out5) -> Scope2/5, Goto4/1
  [CL] -> Mosfet5/1
  Current Measurement/1 -> Max/1, Goto/1
  Bus Selector/3 -> Scope/3  "<Stator current is_a (A)>"
  Permanent Magnet Synchronous Machine/1 -> Bus Selector/1
  [BH] -> Mosfet1/1
  [AH] -> Mosfet6/1
  Bus Selector/4 -> Scope/4  "<Stator current is_b (A)>"
  Gain/1 -> Omega/1, Scope/1  "rotor speed"
  Bus Selector/5 -> Scope/5  "<Stator current is_c (A)>"
  Demux/6 -> [CL]
  Demux/5 -> [CH]
  Demux/4 -> [BL], Scope7/4
  Demux/3 -> Scope7/3, [BH]
  Demux/2 -> Scope7/2, [AL]
  Demux/1 -> Scope7/1, [AH]
  [Vabc] -> Scope4/1  "V"
  Three-Phase V-I Measurement/2 -> Iabc/1, Goto15/1, Scope4/2, Scope3/2  "I"
  Gating Signals/1 -> Demux/1
  Max/1 -> Scope3/1
  Current Measurement1/1 -> Scope3/3
  Constant/1 -> Permanent Magnet Synchronous Machine/1
  connections:
  Mosfet1/RConn1 -- Three-Phase V-I Measurement/LConn2 -- Mosfet4/LConn1
  Mosfet2/RConn1 -- Three-Phase V-I Measurement/LConn3 -- Mosfet5/LConn1
  Mosfet6/RConn1 -- Current Measurement1/LConn1 -- Mosfet3/LConn1
  Mosfet6/LConn1 -- Current Measurement/RConn1 -- Mosfet2/LConn1 -- Mosfet1/LConn1
  Ground/LConn1 -- DC Voltage Source/LConn1 -- Mosfet5/RConn1 -- Mosfet4/RConn1 -- Mosfet3/RConn1
  Three-Phase V-I Measurement/RConn1 -- Permanent Magnet Synchronous Machine/LConn1
  Three-Phase V-I Measurement/RConn2 -- Permanent Magnet Synchronous Machine/LConn2
  Permanent Magnet Synchronous Machine/LConn3 -- Three-Phase V-I Measurement/RConn3
  DC Voltage Source/RConn1 -- Current Measurement/LConn1
  Current Measurement1/RConn1 -- Three-Phase V-I Measurement/LConn1

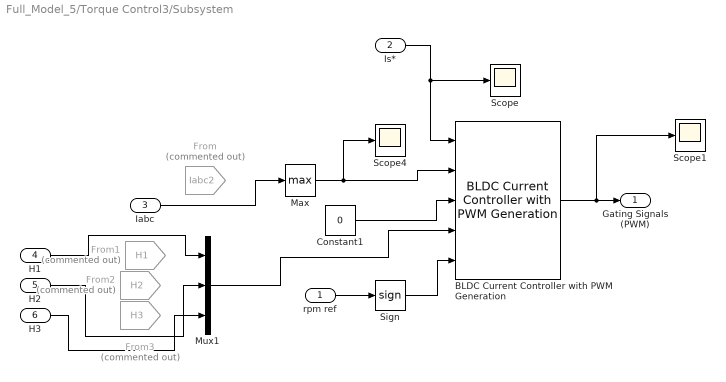
== system Full_Model_5/Torque Control3/Subsystem ==
  rpm ref : Inport
  Is* : Inport  Port=2
  Iabc : Inport  Port=3
  H1 : Inport  Port=4
  H2 : Inport  Port=5
  H3 : Inport  Port=6
  BLDC Current Controller with PWM Generation : peBldcCurrentController/BLDC Current Controller with PWM Generation  Kp=40  Ki=10  Kaw=100  Ts=-1  Tsd=0.001  ActZC=off  CarrCount=Up  Tper=.0001  Tfundamental=.00001
  Constant1 : Constant  Value=0
  From : From  Commented=on  GotoTag=Iabc2  TagVisibility=global
  From1 : From  Commented=on  GotoTag=H1  TagVisibility=global
  From2 : From  Commented=on  GotoTag=H2  TagVisibility=global
  From3 : From  Commented=on  GotoTag=H3  TagVisibility=global
  Max : MinMax  Function=max
  Mux1 : Mux  Inputs=3
  Scope : Scope
  Scope1 : Scope
  Scope4 : Scope
  Sign : Signum
  Gating Signals (PWM) : Outport
  wires:
  H3/1 -> Mux1/3
  H2/1 -> Mux1/2
  H1/1 -> Mux1/1
  Iabc/1 -> Max/1
  Is*/1 -> BLDC Current Controller with PWM Generation/1, Scope/1
  BLDC Current Controller with PWM Generation/1 -> Gating Signals (PWM)/1, Scope1/1
  Max/1 -> Scope4/1, BLDC Current Controller with PWM Generation/2
  Constant1/1 -> BLDC Current Controller with PWM Generation/3
  Sign/1 -> BLDC Current Controller with PWM Generation/5
  Mux1/1 -> BLDC Current Controller with PWM Generation/4
  rpm ref/1 -> Sign/1

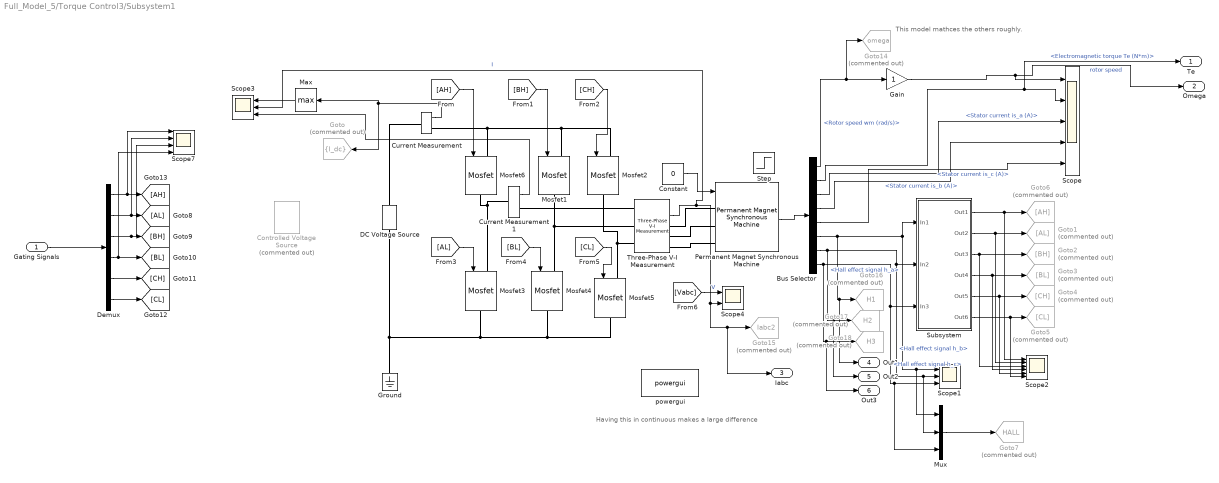
== system Full_Model_5/Torque Control3/Subsystem1 ==
  note: Having this in continuous makes a large difference
  note: This model mathces the others roughly.
  Gating Signals : Inport
  Bus Selector : BusSelector  OutputSignals=Rotor speed wm (rad/s),Electromagnetic torque Te (N*m),Stator current is_a (A),Stator current is_b (A),Stator current is_c (A),Hall effect signal h_a,Hall effect signal h_b,Hall effect signal h_c
  Constant : Constant  Value=0
  Controlled Voltage Source : powerlib/Electrical Sources/Controlled Voltage Source  Commented=on  Initialize=off  Source_Type=DC  Amplitude=24  Phase=0  Frequency=0  Measurements=Voltage
  Current Measurement : powerlib/Measurements/Current Measurement  PhasorSimulation=off  OutputType=Magnitude  PSBequivalent=0
  Current Measurement1 : powerlib/Measurements/Current Measurement  PhasorSimulation=off  OutputType=Complex  PSBequivalent=0
  DC Voltage Source : powerlib/Electrical Sources/DC Voltage Source  Amplitude=24  Measurements=None
  Demux : Demux  Outputs=6
  Gain : Gain
  Goto : Goto  Commented=on  GotoTag=I_dc  TagVisibility=scoped
  Goto1 : Goto  Commented=on  GotoTag=AL
  Goto14 : Goto  Commented=on  GotoTag=omega  TagVisibility=global
  Goto15 : Goto  Commented=on  GotoTag=Iabc2  TagVisibility=global
  Goto16 : Goto  Commented=on  GotoTag=H1  TagVisibility=global
  Goto17 : Goto  Commented=on  GotoTag=H2  TagVisibility=global
  Goto18 : Goto  Commented=on  GotoTag=H3  TagVisibility=global
  Goto2 : Goto  Commented=on  GotoTag=BH
  Goto3 : Goto  Commented=on  GotoTag=BL
  Goto4 : Goto  Commented=on  GotoTag=CH
  Goto5 : Goto  Commented=on  GotoTag=CL
  Goto6 : Goto  Commented=on  GotoTag=AH
  Goto7 : Goto  Commented=on  GotoTag=HALL  TagVisibility=global
  Ground : powerlib/Elements/Ground  LConnTagsString=a
  Max : MinMax  Function=max
  Mosfet{1..6} (6 alike) : powerlib/Power Electronics/Mosfet  Ron=0.1  Lon=0  Rd=0.01  Vfd=0  IC=0  Rs=1e5  Cs=inf  Measurements=off
  Mux : Mux  Inputs=3
  Permanent Magnet Synchronous Machine : powerlib/Machines/Permanent Magnet Synchronous Machine  NbPhases=3  FluxDistribution=Trapezoidal  RotorType=Round  MechanicalLoad=Torque Tm  PresetModel=No  ShowDetailedParameters=on  MeasurementBus=off  Resistance=0.304  Inductance=0.0002315  dqInductances=[8.5e-3,8.5e-3]  La=0.0002315  MachineConstant=Torque Constant (N.m / A_peak)  Flux=0.003258  VoltageCst=5.4588  TorqueCst=0.052128  Flat=120  Mechanical=[1.81e-05 1e-07 8]  PolePairs=4  InitialConditions=[0,0, 0,0]  InitialConditions5ph=[0 0 0 0 0 0]  TsPowergui=0  TsBlock=-1  RefAngle=Aligned with phase A axis (original Park)
      settings: SourceProductName=Simscape Power Systems
  Scope : Scope  NumInputPorts=5
  Scope1 : Scope  NumInputPorts=3
  Scope2 : Scope  NumInputPorts=6
  Scope3 : Scope  NumInputPorts=3
  Scope4 : Scope  NumInputPorts=2
  Scope7 : Scope  NumInputPorts=4
  Step : Step  Time=.1  After=.125  SampleTime=0
  Subsystem : Subsystem
  Three-Phase V-I Measurement : powerlib/Measurements/Three-Phase V-I Measurement  VoltageMeasurement=phase-to-ground  SetLabelV=off  LabelV=Vabc  Vpu=off  VpuLL=off  CurrentMeasurement=yes  SetLabelI=off  LabelI=Iabc  Ipu=off  Pbase=100e6  Vbase=500e3  OutputType=Complex  PhasorSimulation=off  PSBequivalent=0
  powergui : powerlib/powergui  Priority=1  SimulationMode=Continuous  SampleTime=50e-6  frequency=60  Iterations=50  frequencyindice=0  Pbase=100e6  ErrMax=1e-4  UnitsV=kV  UnitsW=MW  buscounter=0  FunctionMessages=off  echomessages=off  EnableUseOfTLC=off  CurrentSourceSwitches=off  DisableSnubberDevices=off  DisableRonSwitches=off  DisableVfSwitches=off  DisplayEquations=off  SolverType=Tustin/Backward Euler (TBE)  Interpol=off  ExternalGateDelay=off  methode=off  Ts=100  x0status=blocks  SPID=on  SwTol=0  HookPort=off  RestoreLinks=warning  ResistiveCurrentMeasurement=off  Frange=[0:2:500]  Ylog=off  Xlog=on  ShowGrid=off  save=off  variable=ZData  structure=0  ZoomFFT=off  StartTime=0.0  cycles=1  DisplayStyle=1  fundamental=60  FreqAxis=off  MaxFrequency=1000  frequencyindicesteady=1  RmsSteady=1  display=off
  Te : Outport
  Omega : Outport  Port=2
  Iabc : Outport  Port=3
  Out1 : Outport  Port=4
  Out2 : Outport  Port=5
  Out3 : Outport  Port=6
  wires:
  Constant/1 -> Permanent Magnet Synchronous Machine/1
  Current Measurement1/1 -> Scope3/3
  Max/1 -> Scope3/1
  Gating Signals/1 -> Demux/1
  Three-Phase V-I Measurement/2 -> Scope3/2, Scope4/2, Goto15/1, Iabc/1  "I"
  [Vabc] -> Scope4/1  "V"
  Demux/1 -> [AH], Scope7/1
  Demux/2 -> [AL], Scope7/2
  Demux/3 -> [BH], Scope7/3
  Demux/4 -> Scope7/4, [BL]
  Demux/5 -> [CH]
  Demux/6 -> [CL]
  Bus Selector/5 -> Scope/5  "<Stator current is_c (A)>"
  Gain/1 -> Scope/1, Omega/1  "rotor speed"
  Bus Selector/4 -> Scope/4  "<Stator current is_b (A)>"
  [AH] -> Mosfet6/1
  [BH] -> Mosfet1/1
  Permanent Magnet Synchronous Machine/1 -> Bus Selector/1
  Bus Selector/3 -> Scope/3  "<Stator current is_a (A)>"
  Current Measurement/1 -> Goto/1, Max/1
  [CL] -> Mosfet5/1
  Subsystem/5(Out5) -> Goto4/1, Scope2/5
  Bus Selector/6 -> Scope1/1, Mux/1, Subsystem/1(In1), Goto16/1, Out1/1  "<Hall effect signal h_a>"
  [BL] -> Mosfet4/1
  [AL] -> Mosfet3/1
  Mux/1 -> Goto7/1
  Bus Selector/7 -> Subsystem/2(In2), Scope1/2, Mux/2, Goto17/1, Out2/1  "<Hall effect signal h_b>"
  Bus Selector/1 -> Gain/1, Goto14/1  "<Rotor speed wm (rad/s)>"
  Subsystem/4(Out4) -> Goto3/1, Scope2/4
  Bus Selector/2 -> Scope/2, Te/1  "<Electromagnetic torque Te (N*m)>"
  Subsystem/3(Out3) -> Goto2/1, Scope2/3
  Subsystem/1(Out1) -> Goto6/1, Scope2/1
  Bus Selector/8 -> Subsystem/3(In3), Scope1/3, Mux/3, Goto18/1, Out3/1  "<Hall effect signal h_c>"
  Subsystem/2(Out2) -> Goto1/1, Scope2/2
  Subsystem/6(Out6) -> Goto5/1, Scope2/6
  [CH] -> Mosfet2/1
  connections:
  Current Measurement1/RConn1 -- Three-Phase V-I Measurement/LConn1
  DC Voltage Source/RConn1 -- Current Measurement/LConn1
  Permanent Magnet Synchronous Machine/LConn3 -- Three-Phase V-I Measurement/RConn3
  Three-Phase V-I Measurement/RConn2 -- Permanent Magnet Synchronous Machine/LConn2
  Three-Phase V-I Measurement/RConn1 -- Permanent Magnet Synchronous Machine/LConn1
  Mosfet3/RConn1 -- Mosfet4/RConn1 -- Mosfet5/RConn1 -- DC Voltage Source/LConn1 -- Ground/LConn1
  Mosfet1/LConn1 -- Mosfet2/LConn1 -- Current Measurement/RConn1 -- Mosfet6/LConn1
  Mosfet3/LConn1 -- Current Measurement1/LConn1 -- Mosfet6/RConn1
  Mosfet5/LConn1 -- Three-Phase V-I Measurement/LConn3 -- Mosfet2/RConn1
  Mosfet4/LConn1 -- Three-Phase V-I Measurement/LConn2 -- Mosfet1/RConn1

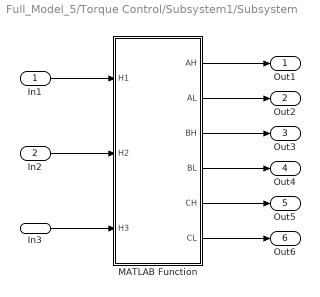
== system Full_Model_5/Torque Control/Subsystem1/Subsystem ==
  In1 : Inport
  In2 : Inport  Port=2
  In3 : Inport  Port=3
  MATLAB Function : MATLAB Function  TreatAsAtomicUnit=on
  Out1 : Outport
  Out2 : Outport  Port=2
  Out3 : Outport  Port=3
  Out4 : Outport  Port=4
  Out5 : Outport  Port=5
  Out6 : Outport  Port=6
  wires:
  In1/1 -> MATLAB Function/1(H1)
  In3/1 -> MATLAB Function/3(H3)
  In2/1 -> MATLAB Function/2(H2)
  MATLAB Function/1(AH) -> Out1/1
  MATLAB Function/2(AL) -> Out2/1
  MATLAB Function/3(BH) -> Out3/1
  MATLAB Function/4(BL) -> Out4/1
  MATLAB Function/6(CL) -> Out6/1
  MATLAB Function/5(CH) -> Out5/1

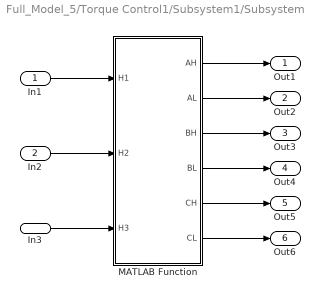
== system Full_Model_5/Torque Control1/Subsystem1/Subsystem ==
  In1 : Inport
  In2 : Inport  Port=2
  In3 : Inport  Port=3
  MATLAB Function : MATLAB Function  TreatAsAtomicUnit=on
  Out1 : Outport
  Out2 : Outport  Port=2
  Out3 : Outport  Port=3
  Out4 : Outport  Port=4
  Out5 : Outport  Port=5
  Out6 : Outport  Port=6
  wires:
  MATLAB Function/5(CH) -> Out5/1
  MATLAB Function/6(CL) -> Out6/1
  MATLAB Function/4(BL) -> Out4/1
  MATLAB Function/3(BH) -> Out3/1
  MATLAB Function/2(AL) -> Out2/1
  MATLAB Function/1(AH) -> Out1/1
  In2/1 -> MATLAB Function/2(H2)
  In3/1 -> MATLAB Function/3(H3)
  In1/1 -> MATLAB Function/1(H1)

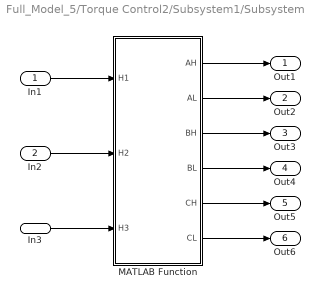
== system Full_Model_5/Torque Control2/Subsystem1/Subsystem ==
  In1 : Inport
  In2 : Inport  Port=2
  In3 : Inport  Port=3
  MATLAB Function : MATLAB Function  TreatAsAtomicUnit=on
  Out1 : Outport
  Out2 : Outport  Port=2
  Out3 : Outport  Port=3
  Out4 : Outport  Port=4
  Out5 : Outport  Port=5
  Out6 : Outport  Port=6
  wires:
  In1/1 -> MATLAB Function/1(H1)
  In3/1 -> MATLAB Function/3(H3)
  In2/1 -> MATLAB Function/2(H2)
  MATLAB Function/1(AH) -> Out1/1
  MATLAB Function/2(AL) -> Out2/1
  MATLAB Function/3(BH) -> Out3/1
  MATLAB Function/4(BL) -> Out4/1
  MATLAB Function/6(CL) -> Out6/1
  MATLAB Function/5(CH) -> Out5/1

== system Full_Model_5/Torque Control3/Subsystem1/Subsystem ==
  In1 : Inport
  In2 : Inport  Port=2
  In3 : Inport  Port=3
  MATLAB Function : MATLAB Function  TreatAsAtomicUnit=on
  Out1 : Outport
  Out2 : Outport  Port=2
  Out3 : Outport  Port=3
  Out4 : Outport  Port=4
  Out5 : Outport  Port=5
  Out6 : Outport  Port=6
  wires:
  MATLAB Function/5(CH) -> Out5/1
  MATLAB Function/6(CL) -> Out6/1
  MATLAB Function/4(BL) -> Out4/1
  MATLAB Function/3(BH) -> Out3/1
  MATLAB Function/2(AL) -> Out2/1
  MATLAB Function/1(AH) -> Out1/1
  In2/1 -> MATLAB Function/2(H2)
  In3/1 -> MATLAB Function/3(H3)
  In1/1 -> MATLAB Function/1(H1)

== matlab function Full_Model_5/Rotation Matrix1 ==
  data: phi input; rot output
function rot = rotation_matrix(phi)
    rot = [cos(phi) -sin(phi) 0; sin(phi) cos(phi) 0; 0 0 1];
end

== matlab function Full_Model_5/Torque Control/Subsystem1/Subsystem/MATLAB Function ==
  data: H1 input; AH output; H2 input; H3 input; AL output; BH output; BL output; CH output; CL output
function [AH, AL, BH, BL, CH, CL] = fcn(H1, H2, H3)
% H1 = int16(H1);
% H2 = int16(H2);
% H3 = int16(H3);
H1
H2
H3
AH = 0;
AL = 0;
BH = 0;
BL = 0;
CH = 0;
CL = 0;
%Rember this does not deal with the PWM signal
if (H1(1) == 1 && H2 == 0 && H3 == 0)
    AH = 1;
    AL = 0;
    BH = 0;
    BL = 1;
    CH = 0;
    CL = 0;
elseif (H1(1) == 1 && H2 == 1 && H3 == 0)
    AH = 1;
    AL = 0;
    BH = 0;
    BL = 0;
    CH = 0;
    CL = 1;
elseif (H1(1) == 0 && H2 == 1 && H3 == 0)
    AH = 0;
    AL = 0;
    BH = 1;
    BL = 0;
    CH = 0;
    CL = 1;
elseif (H1(1) == 0 && H2 == 1 && H3 == 1)
    AH = 0;
    AL = 1;
    BH = 1;
    BL = 0;
    CH = 0;
    CL = 0;
elseif (H1(1) == 0 && H2 == 0 && H3 == 1)
    AH = 0;
    AL = 1;
    BH = 0;
    BL = 0;
    CH = 1;
    CL = 0;
elseif (H1(1) == 1 && H2 == 0 && H3 == 1)
    AH = 0;
    AL = 0;
    BH = 0;
    BL = 1;
    CH = 1;
    CL = 0;
end

== matlab function Full_Model_5/Generate Refrences/Gen Ref Values ==
  data: v input; rx output; t input; rv output; ra output
function [rx, rv, ra] = update_control(v,t)
    rx = [sin(v * t); cos(v * t); v * t];
    rv = v * [cos(v * t); -sin(v * t); v];
    ra = v^2 * [-sin(v * t); -cos(v * t); 0];

%    u = 0.8 * robot_controller.control(pos, vel, rx, rv, ra);
end

== matlab function Full_Model_5/Torque Control1/Subsystem1/Subsystem/MATLAB Function ==
  data: H1 input; AH output; H2 input; H3 input; AL output; BH output; BL output; CH output; CL output
function [AH, AL, BH, BL, CH, CL] = fcn(H1, H2, H3)
% H1 = int16(H1);
% H2 = int16(H2);
% H3 = int16(H3);
H1
H2
H3
AH = 0;
AL = 0;
BH = 0;
BL = 0;
CH = 0;
CL = 0;
%Rember this does not deal with the PWM signal
if (H1(1) == 1 && H2 == 0 && H3 == 0)
    AH = 1;
    AL = 0;
    BH = 0;
    BL = 1;
    CH = 0;
    CL = 0;
elseif (H1(1) == 1 && H2 == 1 && H3 == 0)
    AH = 1;
    AL = 0;
    BH = 0;
    BL = 0;
    CH = 0;
    CL = 1;
elseif (H1(1) == 0 && H2 == 1 && H3 == 0)
    AH = 0;
    AL = 0;
    BH = 1;
    BL = 0;
    CH = 0;
    CL = 1;
elseif (H1(1) == 0 && H2 == 1 && H3 == 1)
    AH = 0;
    AL = 1;
    BH = 1;
    BL = 0;
    CH = 0;
    CL = 0;
elseif (H1(1) == 0 && H2 == 0 && H3 == 1)
    AH = 0;
    AL = 1;
    BH = 0;
    BL = 0;
    CH = 1;
    CL = 0;
elseif (H1(1) == 1 && H2 == 0 && H3 == 1)
    AH = 0;
    AL = 0;
    BH = 0;
    BL = 1;
    CH = 1;
    CL = 0;
end

== matlab function Full_Model_5/Torque Control2/Subsystem1/Subsystem/MATLAB Function ==
  data: H1 input; AH output; H2 input; H3 input; AL output; BH output; BL output; CH output; CL output
function [AH, AL, BH, BL, CH, CL] = fcn(H1, H2, H3)
% H1 = int16(H1);
% H2 = int16(H2);
% H3 = int16(H3);
H1
H2
H3
AH = 0;
AL = 0;
BH = 0;
BL = 0;
CH = 0;
CL = 0;
%Rember this does not deal with the PWM signal
if (H1(1) == 1 && H2 == 0 && H3 == 0)
    AH = 1;
    AL = 0;
    BH = 0;
    BL = 1;
    CH = 0;
    CL = 0;
elseif (H1(1) == 1 && H2 == 1 && H3 == 0)
    AH = 1;
    AL = 0;
    BH = 0;
    BL = 0;
    CH = 0;
    CL = 1;
elseif (H1(1) == 0 && H2 == 1 && H3 == 0)
    AH = 0;
    AL = 0;
    BH = 1;
    BL = 0;
    CH = 0;
    CL = 1;
elseif (H1(1) == 0 && H2 == 1 && H3 == 1)
    AH = 0;
    AL = 1;
    BH = 1;
    BL = 0;
    CH = 0;
    CL = 0;
elseif (H1(1) == 0 && H2 == 0 && H3 == 1)
    AH = 0;
    AL = 1;
    BH = 0;
    BL = 0;
    CH = 1;
    CL = 0;
elseif (H1(1) == 1 && H2 == 0 && H3 == 1)
    AH = 0;
    AL = 0;
    BH = 0;
    BL = 1;
    CH = 1;
    CL = 0;
end

== matlab function Full_Model_5/Torque Control3/Subsystem1/Subsystem/MATLAB Function ==
  data: H1 input; AH output; H2 input; H3 input; AL output; BH output; BL output; CH output; CL output
function [AH, AL, BH, BL, CH, CL] = fcn(H1, H2, H3)
% H1 = int16(H1);
% H2 = int16(H2);
% H3 = int16(H3);
H1
H2
H3
AH = 0;
AL = 0;
BH = 0;
BL = 0;
CH = 0;
CL = 0;
%Rember this does not deal with the PWM signal
if (H1(1) == 1 && H2 == 0 && H3 == 0)
    AH = 1;
    AL = 0;
    BH = 0;
    BL = 1;
    CH = 0;
    CL = 0;
elseif (H1(1) == 1 && H2 == 1 && H3 == 0)
    AH = 1;
    AL = 0;
    BH = 0;
    BL = 0;
    CH = 0;
    CL = 1;
elseif (H1(1) == 0 && H2 == 1 && H3 == 0)
    AH = 0;
    AL = 0;
    BH = 1;
    BL = 0;
    CH = 0;
    CL = 1;
elseif (H1(1) == 0 && H2 == 1 && H3 == 1)
    AH = 0;
    AL = 1;
    BH = 1;
    BL = 0;
    CH = 0;
    CL = 0;
elseif (H1(1) == 0 && H2 == 0 && H3 == 1)
    AH = 0;
    AL = 1;
    BH = 0;
    BL = 0;
    CH = 1;
    CL = 0;
elseif (H1(1) == 1 && H2 == 0 && H3 == 1)
    AH = 0;
    AL = 0;
    BH = 0;
    BL = 1;
    CH = 1;
    CL = 0;
end
